simulink model "pilot_data_generator"  (R2020a)
settings: Solver=FixedStepAuto  StartTime=0.0  StopTime=90  FixedStep=1/100  RelTol=1e-3
values from neighbouring files (symbols this model uses):
  K_r = 0.0    (= 0)    [simulate_pilot_actual_parameters.m]
  K_s = 0.2865    [generate_transfer_functions.m]    (also in generate_transfer_functions_actual_parameters.m)
  Mot_Resp = 0    [calculate_remnant_parameters.m]    (also in pilot_model.m = false; plot_box_parameters.m = false; save_remnant_parameters.m = false; simulate_pilot_actual_parameters.m = false)
libraries: cstblocks x4
settings Model: Creator=tijn-  LastModifiedBy=tijn-

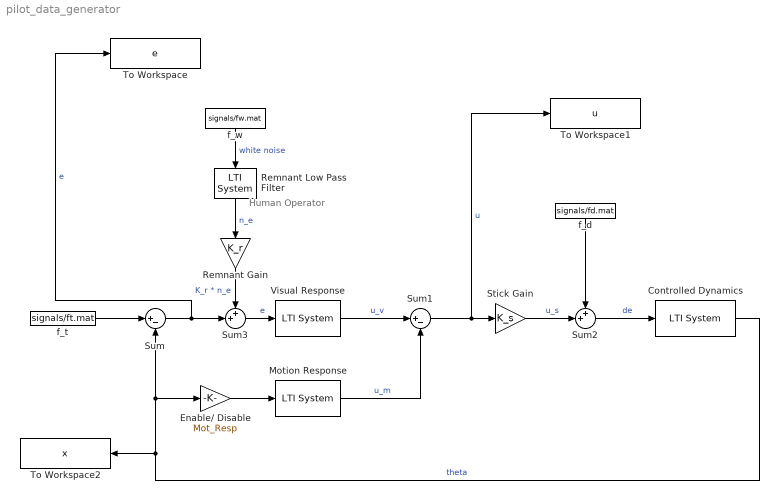
== system pilot_data_generator ==
  note: Human Operator
  Controlled Dynamics : cstblocks/LTI System  sys=H_theta_de  IC=[]
  Enable/ Disable : Gain  Gain=Mot_Resp
  Motion Response : cstblocks/LTI System  sys=H_p_m  IC=[]
  Remnant Gain : Gain  Gain=K_r
  Remnant Low Pass Filter : cstblocks/LTI System  sys=H_n  IC=[]
  "Stick Gain " : Gain  Gain=K_s
  Sum : Sum  Inputs=|+-
  Sum1 : Sum  Inputs=|+-
  Sum2 : Sum  Inputs=++|
  Sum3 : Sum  Inputs=++|
  To Workspace : ToWorkspace  VariableName=e  SampleTime=-1
  To Workspace1 : ToWorkspace  VariableName=u  SampleTime=-1
  To Workspace2 : ToWorkspace  VariableName=x  SampleTime=-1
  Visual Response : cstblocks/LTI System  sys=H_p_v  IC=[]
  f_d : FromFile  FileName=signals/fd.mat  SampleTime=0
  f_t : FromFile  FileName=signals/ft.mat  SampleTime=0
  f_w : FromFile  FileName=signals/fw.mat  SampleTime=0
  wires:
  Sum/1 -> Sum3/2, To Workspace/1  "e"
  Sum1/1 -> To Workspace1/1, "Stick Gain "/1  "u"
  "Stick Gain "/1 -> Sum2/2  "u_s"
  f_d/1 -> Sum2/1
  Sum2/1 -> Controlled Dynamics/1  "de"
  Controlled Dynamics/1 -> To Workspace2/1, Sum/2, Enable/ Disable/1  "theta"
  Enable/ Disable/1 -> Motion Response/1
  Visual Response/1 -> Sum1/1  "u_v"
  Motion Response/1 -> Sum1/2  "u_m"
  f_t/1 -> Sum/1
  f_w/1 -> Remnant Low Pass Filter/1  "white noise"
  Remnant Low Pass Filter/1 -> Remnant Gain/1  "n_e"
  Remnant Gain/1 -> Sum3/1  "K_r * n_e"
  Sum3/1 -> Visual Response/1  "e"
